simulink model "BEMS_system"  (R2020a)
settings: Solver=VariableStepAuto  StartTime=0.0  StopTime=10.0  RelTol=1e-3
undefined symbols (not defined in the file): sigbuilder_block
settings Model: NumberOfSteps=10  Creator=LOGID0142  LastModifiedBy=ramachandran

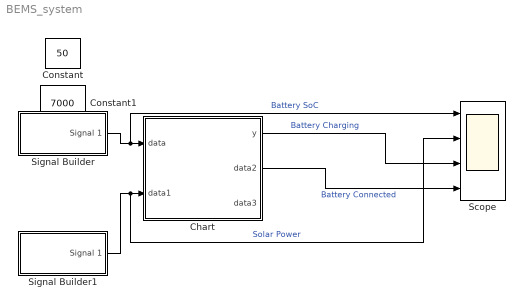
== system BEMS_system ==
  Chart : Stateflow chart  TreatAsAtomicUnit=on
  Constant : Constant  Value=50
  Constant1 : Constant  Value=7000
  Scope : Scope  NumInputPorts=4
  Signal Builder : Subsystem  Tag=STV Subsys  LoadFcn=sigbuilder_block('load',[437.6 153 550.4 359.25 ]);  StartFcn=sigbuilder_block('start');  StopFcn=sigbuilder_block('stop');  ClipboardFcn=sigbuilder_block('clipboard');  mask(Sigbuilder block){tuvar=[0:10]}
      mask help: Simulink:masks:SigbuilderBlock_MD
      mask init:
      | if ~strcmp(get_param(bdroot(gcbh),'SimulationStatus'),'stopped') tuvar = sigbuilder_block('maskInit'); end
      settings: CopyFcn=sigbuilder_block('copy');  DeleteFcn=sigbuilder_block('delete');  ModelCloseFcn=sigbuilder_block('modelClose');  PreSaveFcn=sigbuilder_block('preSave');  PauseFcn=sigbuilder_block('pause');  ContinueFcn=sigbuilder_block('continue');  NameChangeFcn=sigbuilder_block('namechange');  OpenFcn=sigbuilder_block('open',[437.6 199.2 550.4 400 ]);  CloseFcn=sigbuilder_block('close');
      mask Display: plot(0, 0, 100, 100,[2, 2, 32, 32, 2], [68, 8, 8, 68, 68],[32, 2], [38, 38], [32, 19, 2],[53, 60, 44], [32, 17, 17, 2],[16, 16, 31, 31]);txt = getActiveGroup(gcbh);text(2, 100, txt,'verticalAlignment', 'top');
  Signal Builder1 : Subsystem  Tag=STV Subsys  LoadFcn=sigbuilder_block('load');  StartFcn=sigbuilder_block('start');  StopFcn=sigbuilder_block('stop');  ClipboardFcn=sigbuilder_block('clipboard');  mask(Sigbuilder block){tuvar=[0:10]}
      mask help: Simulink:masks:SigbuilderBlock_MD
      mask init:
      | if ~strcmp(get_param(bdroot(gcbh),'SimulationStatus'),'stopped') tuvar = sigbuilder_block('maskInit'); end
      settings: CopyFcn=sigbuilder_block('copy');  DeleteFcn=sigbuilder_block('delete');  ModelCloseFcn=sigbuilder_block('modelClose');  PreSaveFcn=sigbuilder_block('preSave');  PauseFcn=sigbuilder_block('pause');  ContinueFcn=sigbuilder_block('continue');  NameChangeFcn=sigbuilder_block('namechange');  OpenFcn=sigbuilder_block('open',[437.6 153 550.4 359.25 ]);  CloseFcn=sigbuilder_block('close');
      mask Display: plot(0, 0, 100, 100,[2, 2, 32, 32, 2], [68, 8, 8, 68, 68],[32, 2], [38, 38], [32, 19, 2],[53, 60, 44], [32, 17, 17, 2],[16, 16, 31, 31]);txt = getActiveGroup(gcbh);text(2, 100, txt,'verticalAlignment', 'top');
  wires:
  Signal Builder/1(Signal 1) -> Scope/1, Chart/1(data)  "Battery SoC"
  Signal Builder1/1(Signal 1) -> Scope/2, Chart/2(data1)  "Solar Power"
  Chart/1(y) -> Scope/3  "Battery Charging"
  Chart/2(data2) -> Scope/4  "Battery Connected"

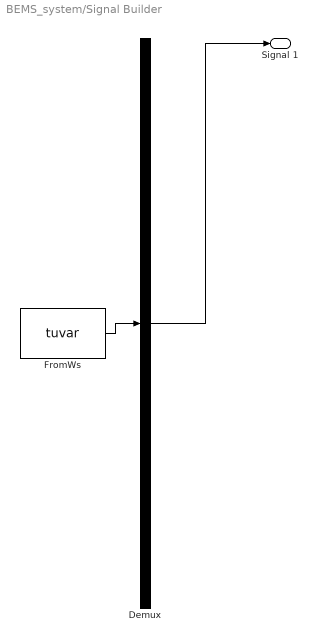
== system BEMS_system/Signal Builder ==
  Demux : Demux  Tag=STV Demux  Outputs=1
      settings: DisplayOption=none
  FromWs : FromWorkspace  Tag=STV FromWs  VariableName=tuvar
      SigBuilderData=|
      | common.afterFinalStr = 'Extrapolate'
      | common.sampleTime = 0
      | dataSet.timeRange = [0 10]
      | dataSet.name = 'Group 1'
      | sbobj.Groups.Name = 'Group 1'
      | sbobj.Groups.Signals.Name = 'Signal 1'
      | sbobj.Groups.Signals.XData = [0 2 2 4 4 6 6 8 8 9.06 9.06 10]
      | sbobj.Groups.Signals.YData = [80 80 67.5 67.5 6 6 44.5 44.5 61.5 61.5 3.5 3.5]
  Signal 1 : Outport  Tag=STV Outport
  wires:
  Demux/1 -> Signal 1/1
  FromWs/1 -> Demux/1

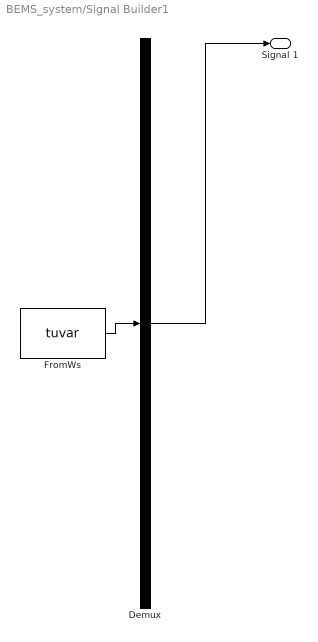
== system BEMS_system/Signal Builder1 ==
  Demux : Demux  Tag=STV Demux  Outputs=1
      settings: DisplayOption=none
  FromWs : FromWorkspace  Tag=STV FromWs  VariableName=tuvar
      SigBuilderData=|
      | common.afterFinalStr = 'Extrapolate'
      | common.sampleTime = 0
      | dataSet.timeRange = [0 10]
      | dataSet.name = 'Group 1'
      | sbobj.Groups.Name = 'Group 1'
      | sbobj.Groups.Signals.Name = 'Signal 1'
      | sbobj.Groups.Signals.XData = [0 1.98 1.98 4 4 6 6 8.04 8.04 9 9 10]
      | sbobj.Groups.Signals.YData = [10000 10000 6600 6600 3200 3200 800 800 9150 9150 750 750]
  Signal 1 : Outport  Tag=STV Outport
  wires:
  FromWs/1 -> Demux/1
  Demux/1 -> Signal 1/1

== stateflow chart BEMS_system/Chart ==
  state Mode_1
    y=1;
    data2=1;
    data3=0;
  state Input_State
  state PV_power_above_5000W
  note: for input
  state Mode_6
    y=1;
    data2=0;
    data3=0;
  state Mode_2
    y=1;
    data2=0;
    data3=0;
  state PV_power_below_5000W
  state Mode_3
    y=1;
    data2=0;
    data3=1;
  state Mode_5
    y=0;
    data2=0;
    data3=0;
  state Mode_4
    y=0;
    data2=0;
    data3=1;
  (default) -> Input_State
  PV_power_above_5000W -> Mode_1 [order 1] : [ data < 80 & data1 > 5000]
  PV_power_above_5000W -> Input_State [order 2] : [ data1 < 5000 ]
  PV_power_below_5000W -> Input_State [order 1] : [ data1 > 5000]
  Input_State -> PV_power_above_5000W [order 1] : [ data1 > 5000]
  Mode_1 -> PV_power_above_5000W [order 1] : [ data > 80]
  Input_State -> PV_power_below_5000W [order 2] : [ data1 < 5000]
  Input_State -> Mode_6 [order 3]
  PV_power_above_5000W -> Mode_2 [order 3] : [ data > 80]
  Mode_2 -> PV_power_above_5000W [order 1] : [ data < 80]
  Mode_2 -> PV_power_above_5000W [order 2] : [ data1 < 5000]
  Mode_1 -> PV_power_above_5000W [order 2] : [ data1 < 5000]
  PV_power_below_5000W -> Mode_3 [order 2] : [ data > 20]
  Mode_3 -> PV_power_below_5000W [order 1] : [ data < 20 & data1 < 2000]
  Mode_5 -> PV_power_below_5000W : [data > 20]
  PV_power_below_5000W -> Mode_3 [order 4] : [ data1 > 2000 & data1 < 5000]
  PV_power_below_5000W -> Mode_5 [order 3] : [ data < 20 & data1 < 2000]
  Mode_3 -> PV_power_below_5000W [order 3] : [ data > 20 & data1 > 5000]
  Mode_4 -> Mode_3 [order 1] : [data1 > 5000]
  Mode_4 -> Mode_3 [order 2] : [ data > 20 & data1 > 2000]
  Mode_3 -> Mode_4 [order 2] : [ data > 20 & data1 < 2000]
  data: data input; y output; data1 input; data2 output; data3 output
